simulink model "BodyHalf"  (R2021b)
settings: Solver=VariableStepAuto  StartTime=0.0  StopTime=10.0  RelTol=1e-3
values from neighbouring files (symbols this model uses):
  a = b    (= 1.4)    [CarQuarterParam.m]
  b = 1.4    [CarQuarterParam.m]
  I = 600    [CarQuarterParam.m]
  M1 = 500    [CarQuarterParam.m]
settings Model: Creator=Reece Bell  LastModifiedBy=reece
settings SolverCC: AlgebraicLoopSolver=TrustRegion
settings DataIOCC: ReturnWorkspaceOutputs=off
settings DebuggingCC: SFMachineParentedDataDiag=warning  ArithmeticOperatorsInVariantConditions=warning
settings SFSimCC: CustomCodeUndefinedFunction=UseInterfaceOnly

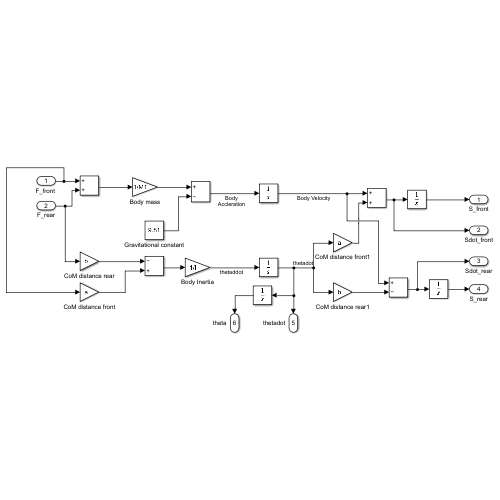
[thumbnail: Simulink's stored preview of the top-level diagram]
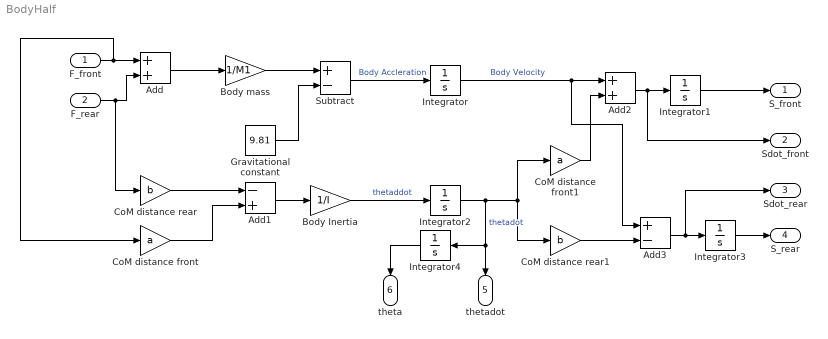
== system BodyHalf ==
  "F_front " : Inport
  F_rear : Inport  Port=2
  Add : Sum
  Add1 : Sum  Inputs=-+
  Add2 : Sum
  Add3 : Sum  Inputs=+-
  Body Inertia : Gain  Gain=1/I
  "Body mass " : Gain  Gain=1/M1
  CoM distance front : Gain  Gain=a
  CoM distance front1 : Gain  Gain=a
  CoM distance rear : Gain  Gain=b
  CoM distance rear1 : Gain  Gain=b
  Gravitational constant : Constant  Value=9.81
  Integrator{,1..4} (5 alike) : Integrator
  Subtract : Sum  Inputs=+-
  S_front : Outport  VectorParamsAs1DForOutWhenUnconnected=off
  Sdot_front : Outport  Port=2  VectorParamsAs1DForOutWhenUnconnected=off
  Sdot_rear : Outport  Port=3  VectorParamsAs1DForOutWhenUnconnected=off
  S_rear : Outport  Port=4  VectorParamsAs1DForOutWhenUnconnected=off
  thetadot : Outport  Port=5
  theta : Outport  Port=6
  wires:
  Subtract/1 -> Integrator/1  "Body Accleration"
  Integrator/1 -> Add3/1, Add2/1  "Body Velocity"
  F_rear/1 -> CoM distance rear/1, Add/2
  "F_front "/1 -> Add/1, CoM distance front/1
  Add/1 -> "Body mass "/1
  "Body mass "/1 -> Subtract/1
  Gravitational constant/1 -> Subtract/2
  Body Inertia/1 -> Integrator2/1  "thetaddot"
  Integrator2/1 -> Integrator4/1, thetadot/1, CoM distance rear1/1, CoM distance front1/1  "thetadot"
  CoM distance front/1 -> Add1/2
  CoM distance rear/1 -> Add1/1
  Add1/1 -> Body Inertia/1
  CoM distance front1/1 -> Add2/2
  Add2/1 -> Sdot_front/1, Integrator1/1
  CoM distance rear1/1 -> Add3/2
  Add3/1 -> Sdot_rear/1, Integrator3/1
  Integrator1/1 -> S_front/1
  Integrator3/1 -> S_rear/1
  Integrator4/1 -> theta/1
